simulink model "modelo_f_NIVEL_2_DISCRETIZADO"  (R2023a)
settings: Solver=ode15s  StartTime=0.0  StopTime=60  FixedStep=T_s  RelTol=1e-3
InitFcn:
  | clc
  | clear
  | close all
  | parametros
  | gain_CL
  | calculo_observador_carro
  | calculo_observador_izaje
undefined symbols (not defined in the file): b_cx, b_cy, b_ha, b_hb, b_hd, b_hm, b_t, b_ta, b_tb, b_td, b_tm, b_tw, b_wu, carro_FC_safety_margin, g, H_c, i_h, i_t, izaje_FC_safety_margin, J_hd_hEb, J_hm_hb, J_td, J_tm_tb, K_cy, k_hsa, k_hsia, k_tsa, k_tsia, K_tw, k_wu, l_h_max, l_h_maxE, l_h_min, l_h_minE, Lh, Lt, M_cmax, M_cmin, M_s, M_t, M_tEq, r_hd, r_td, T_hbMax, T_hEbMax, T_hmMax, T_s, T_tbMax, T_tmMax, tau_tm, theta_hm0, theta_tm0, v_h_max_noload, v_lx0, v_ly0, v_t0, v_t_max, W_c, w_hm0, w_hm_min_BRK ... (+14)
libraries: dspsigops x1, simulink x1
(part 2 of 2)

== matlab function modelo_f_NIVEL_2_DISCRETIZADO/MATLAB Function1 ==
  data: t input; l_h_star output; t_inicio input; l_inicial input; l_final input; masa_total input; dl_h_star output; ddl_h_star output
function [l_h_star, dl_h_star, ddl_h_star] = generador_trayectoria_izaje(t, t_inicio, l_inicial, l_final, masa_total)
    % ---------------------------------------------------------------------
    % CONSTANTES FISICAS Y OPERATIVAS DE IZAJE
    % ---------------------------------------------------------------------
    g = 9.80665;               
    P_const = 956150;          
    v_max_absoluta = 3.0;      
    a_max_limite = 0.75;       
    
    % Operación a potencia constante según carga actual
    v_potencia = P_const / (masa_total * g);
    v_max_limite = min(v_max_absoluta, v_potencia);
    
    if t < t_inicio
        l_h_star = l_inicial;
        dl_h_star = 0;
        ddl_h_star = 0;
        return;
    end
    
    t_eff = t - t_inicio;
    D = abs(l_final - l_inicial);
    dir = sign(l_final - l_inicial); 
    
    if D == 0
        l_h_star = l_inicial;
        dl_h_star = 0;
        ddl_h_star = 0;
        return;
    end
    
    % ---------------------------------------------------------------------
    % CALCULO DEL PERFIL CINEMATICO (Curva S con Jerk continuo: 1 - cos)
    % ---------------------------------------------------------------------
    % Tiempo para alcanzar la velocidad máxima con este perfil
    t_a = 2 * v_max_limite / a_max_limite;
    d_a = v_max_limite * t_a / 2;
    
    if 2 * d_a >= D
        % Perfil sin crucero (Triangular ultra-suavizado)
        v_pico = sqrt((D * a_max_limite) / 2);
        t_a = 2 * v_pico / a_max_limite;
        t_crucero = 0;
        v_crucero = v_pico;
        d_crucero = 0;
        d_a = D / 2;
    else
        % Perfil Trapezoidal ultra-suavizado
        v_crucero = v_max_limite;
        d_crucero = D - 2 * d_a;
        t_crucero = d_crucero / v_crucero;
    end
    
    t_total = 2 * t_a + t_crucero;
    
    % ---------------------------------------------------------------------
    % EVALUACION INSTANTANEA
    % ---------------------------------------------------------------------
    if t_eff < t_a
        % Fase 1: Aceleración Suave (Perfil campana 1-cos)
        ddl_h_star = (a_max_limite / 2) * (1 - cos(2 * pi * t_eff / t_a)) * dir;
        dl_h_star = (a_max_limite / 2) * (t_eff - (t_a / (2 * pi)) * sin(2 * pi * t_eff / t_a)) * dir;
        l_h_star = l_inicial + (a_max_limite / 2) * ((t_eff^2 / 2) + (t_a^2 / (4 * pi^2)) * (cos(2 * pi * t_eff / t_a) - 1)) * dir;
        
    elseif t_eff < (t_a + t_crucero)
        % Fase 2: Velocidad Constante de Crucero
        t_fase2 = t_eff - t_a;
        ddl_h_star = 0;
        dl_h_star = v_crucero * dir;
        l_h_star = l_inicial + d_a * dir + v_crucero * t_fase2 * dir;
        
    elseif t_eff < t_total
        % Fase 3: Desaceleración Suave (Campana invertida 1-cos)
        t_fase3 = t_eff - (t_a + t_crucero);
        ddl_h_star = -(a_max_limite / 2) * (1 - cos(2 * pi * t_fase3 / t_a)) * dir;
        dl_h_star = (v_crucero - (a_max_limite / 2) * (t_fase3 - (t_a / (2 * pi)) * sin(2 * pi * t_fase3 / t_a))) * dir;
        
        d_recorrida_fase3 = v_crucero * t_fase3 - (a_max_limite / 2) * ((t_fase3^2 / 2) + (t_a^2 / (4 * pi^2)) * (cos(2 * pi * t_fase3 / t_a) - 1));
        l_h_star = l_inicial + (d_a + d_crucero + d_recorrida_fase3) * dir;
        
    else
        % Fase 4: Posición final alcanzada
        l_h_star = l_final;
        dl_h_star = 0;
        ddl_h_star = 0;
    end
end

== matlab function modelo_f_NIVEL_2_DISCRETIZADO/Nivel 2/Subsistema físico/MATLAB Function ==
  data: x_t_min input; y_c0_contacto output; x_t_max input; Y_sb input; W_c input; y_h_min input; H_c input; x_lidar_offset input; x_l input; TLK input; y_c0_lidar output
function [y_c0_contacto, y_c0_lidar] = perfil_suelo(x_t_min, x_t_max, Y_sb, W_c, y_h_min, H_c, x_lidar_offset, x_l, TLK)

persistent n_containers x_grid tlk_prev

%% Inicialización de perfil

if isempty(n_containers)
    x_grid       = x_t_min : W_c : x_t_max;
    n_containers = zeros(1, length(x_grid));
    tlk_prev     = false;
end

%% Índice más cercano a x_l

[~, idx] = min(abs(x_grid - x_l));

%% Extracción y depósito de contenedores

flanco_bajada = (tlk_prev == 1) && (TLK == 0);
flanco_subida = (tlk_prev == 0) && (TLK == 1);

if flanco_bajada
    n_containers(idx) = n_containers(idx) + 1;
elseif flanco_subida
    n_containers(idx) = max(0, n_containers(idx) - 1);
end

tlk_prev = TLK;

%% Altura fija según zona
if x_l < -W_c/2
    y_fijo = 0;
elseif x_l >= -W_c/2 && x_l <= W_c/2
    y_fijo = Y_sb;
else
    y_fijo = y_h_min;
end

%% Altura total
y_c0_contacto = y_fijo + n_containers(idx) * H_c;

%% Lectura de lidar
x_laser = x_l + x_lidar_offset; % Definimos la posición exacta del láser
[~, idx_lidar] = min(abs(x_grid - x_laser));

% Ahora evaluamos las zonas usando la visión del láser, no de la carga
if x_laser < -W_c/2
    y_fijo_lidar = 0;
elseif x_laser >= -W_c/2 && x_laser <= W_c/2
    y_fijo_lidar = Y_sb;
else
    y_fijo_lidar = y_h_min;
end

y_c0_lidar = y_fijo_lidar + n_containers(idx_lidar) * H_c;

== stateflow chart modelo_f_NIVEL_2_DISCRETIZADO/Chart ==
  state Supervisory_Control
    state ON
      state BRK_Logic [parallel]
        settings: executionOrder=1
        state BRK_t_Logic [parallel]
          settings: executionOrder=1
          state BRK_t_Closed
            entry:
            BRK_t = false;
          state BRK_t_Opened
            entry:
            BRK_t = true;
          (default) -> BRK_t_Closed
          BRK_t_Opened -> BRK_t_Closed : [(~cmd_BRK_t && abs(w_tm_estimada) < w_tm_min_BRK) || FC_carro_min || FC_carro_max]
          BRK_t_Closed -> BRK_t_Opened : [cmd_BRK_t && ~(FC_carro_max || FC_carro_min)]
        state BRK_h_Logic [parallel]
          settings: executionOrder=2
          state BRK_h_Closed
            entry:
            BRK_h = false;
          state BRK_h_Opened
            entry:
            BRK_h = true;
          (default) -> BRK_h_Closed
          BRK_h_Opened -> BRK_h_Closed : [(~cmd_BRK_h && abs(w_hm_estimada) < w_hm_min_BRK) || FC_izaje_min || FC_izaje_max]
          BRK_h_Closed -> BRK_h_Opened : [cmd_BRK_h && ~(FC_izaje_max || FC_izaje_min)]
      state TLK_Logic [parallel]
        settings: executionOrder=2
        state Init
        state TLK_Opened
          entry:
          TLK = false;
        state TLK_Closed
          entry:
          TLK = true;
        (default) -> Init
        Init -> TLK_Closed [order 1] : [TLK]
        Init -> TLK_Opened [order 2] : [~TLK]
        TLK_Opened -> TLK_Closed : [cmd_TLK && abs(F_hw_sensor) <= 0]
        TLK_Closed -> TLK_Opened : [~cmd_TLK && abs(F_hw_sensor) <= 0]
      state Sway_Control_Mode [parallel]
        settings: executionOrder=3
        state Sway_Control_ON
          entry:
          sway_ctr_enable = true;
        state Sway_Control_OFF
          entry:
          sway_ctr_enable = false;
        (default) -> Sway_Control_ON
        Sway_Control_ON -> Sway_Control_OFF : [~cmd_sway_ctr]
        Sway_Control_OFF -> Sway_Control_ON : [cmd_sway_ctr && operation_mode == false]
      state Heartbeat_Generator [parallel]
        settings: executionOrder=4
        state Heartbeat_High
          entry:
          heartbeat = true;
        state Heartbeat_Low
          entry:
          heartbeat = false;
        (default) -> Heartbeat_High
        Heartbeat_Low -> Heartbeat_High : after(200, msec)
        Heartbeat_High -> Heartbeat_Low : after(200, msec)
      state Limit_Switch [parallel]
        during:
        force_manual_mode = FC_t_min_alarm || FC_t_max_alarm || FC_h_min_alarm || FC_h_max_alarm;
        settings: executionOrder=5
        state Trolley_Min_Logic [parallel]
          settings: executionOrder=1
          state FC_t_Min_High
            entry:
            FC_t_min_alarm = true;
          state FC_t_Min_Low
            entry:
            FC_t_min_alarm = false;
          (default) -> FC_t_Min_Low
          FC_t_Min_Low -> FC_t_Min_High : [FC_carro_min]
          FC_t_Min_High -> FC_t_Min_Low : [cmd_carro_FC_ack && x_td_sensor >= x_t_min + carro_FC_safety_margin]
        state Trolley_Max_Logic [parallel]
          settings: executionOrder=2
          state FC_t_Max_High
            entry:
            FC_t_max_alarm = true;
          state FC_t_Max_Low
            entry:
            FC_t_max_alarm = false;
          (default) -> FC_t_Max_Low
          FC_t_Max_Low -> FC_t_Max_High : [FC_carro_max]
          FC_t_Max_High -> FC_t_Max_Low : [cmd_carro_FC_ack && x_td_sensor <= x_t_max - carro_FC_safety_margin]
        state Hoist_Min_Logic [parallel]
          settings: executionOrder=3
          state FC_h_Min_High
            entry:
            FC_h_min_alarm = true;
            dl_h_ref = 0;
          state FC_h_Min_Low
            entry:
            FC_h_min_alarm = false;
          (default) -> FC_h_Min_Low
          FC_h_Min_Low -> FC_h_Min_High : [FC_izaje_min]
          FC_h_Min_High -> FC_h_Min_Low : [cmd_izaje_FC_ack && l_h_sensor >= l_h_minE + izaje_FC_safety_margin]
        state Hoist_Max_Logic [parallel]
          settings: executionOrder=4
          state FC_h_Max_Low
            entry:
            FC_h_max_alarm = false;
          state FC_h_Max_High
            entry:
            FC_h_max_alarm = true;
          (default) -> FC_h_Max_Low
          FC_h_Max_Low -> FC_h_Max_High : [FC_izaje_max]
          FC_h_Max_High -> FC_h_Max_Low : [cmd_izaje_FC_ack && l_h_sensor <= l_h_max - izaje_FC_safety_margin]
      state Lidar_Map [parallel]
        entry:
        y(:) = 0;
        during:
        x_idx = round((x_td_sensor - x_t_min) / 0.01) + 1;
        x_idx = max(1, min(length(y), x_idx));
        y(x_idx) = y_c0_lidar;
        settings: executionOrder=6
      state Mode [parallel]
        settings: executionOrder=7
        state Automatic
          during:
          v_t_ref = 1.0;
          operation_mode = true
        state Manual
          during:
          v_t_ref = 0;
        (default) -> Automatic
        Automatic -> Manual : [force_manual_mode]
        Manual -> Automatic : [1==0]
    state OFF
      entry:
      BRK_h = false;
      BRK_t = false;
      TLK = false;
      v_t_ref = 0.0;
      dl_h_ref = 0.0;
      sway_ctr_enable = false;
      FC_t_min_alarm = false;
      FC_t_max_alarm = false;
      FC_h_min_alarm = false;
      FC_h_max_alarm = false;
      force_manual_mode = false;
      sway_ctr_enable = false;
      heartbeat = false;
      operation_mode = true;
    (default) -> OFF
    OFF -> ON : [P_APN]
    ON -> OFF : [~P_APN]
  (default) -> Supervisory_Control
  data: FCE_izaje_min input boolean size=1; BRK_t output boolean size=1; v_t_ref output double size=1; cmd_TLK output; BRK_h output boolean size=1; x_td_sensor input; theta_tm_sensor input; l_h_sensor input; theta_hm_sensor input; theta_l_sensor input; w_l_sensor input; w_tm_estimada input; w_hm_estimada input; y_c0_lidar input; P_APN input; P_E input boolean; cmd_carro_FC_ack input; cmd_sway_ctr input; cmd_izaje_FC_ack input; FCE_carro_min input boolean; FCE_carro_max input boolean size=1; FC_izaje_min input; FC_izaje_max input; FCE_izaje_max input boolean; sobrevelocidad_carro input; sobrevelocidad_izaje_noload input; FC_carro_max input; FC_carro_min input; cmd_TLK input; cmd_BRK_h input; cmd_BRK_t input; F_hw_sensor input; w_hm_min_BRK parameter; w_tm_min_BRK parameter; sway_ctr_enable output boolean size=1; dl_h_ref output double size=1; FC_h_max_alarm local; FC_h_min_alarm local; FC_t_max_alarm local; FC_t_min_alarm local; TLK local; dx_grid local; force_manual_mode local; n_grid local; x_idx local; heartbeat output boolean size=1; operation_mode local; y local double size=LIDAR_GRID_SIZE; izaje_FC_safety_margin parameter; carro_FC_safety_margin parameter; l_h_max parameter; x_t_max parameter; x_t_min parameter; l_h_minE parameter
